simulink model "quhua"  (Simulink 6.3)
settings: Solver=ode45  StartTime=0.0  StopTime=0.08  RelTol=1e-3
settings Model: LastModifiedBy=Administrator

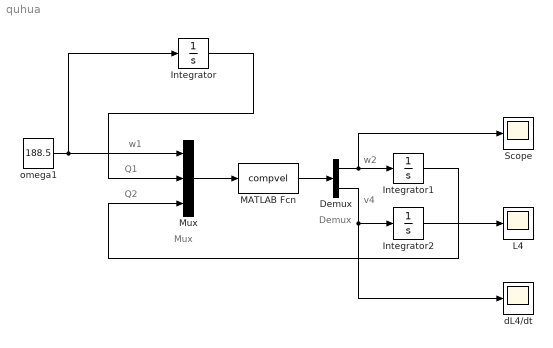
== system quhua ==
  note: Mux
  note: Demux
  note: w1
  note: Q1
  note: Q2
  note: w2
  note: v4
  Demux : Demux  Outputs=2
  Integrator : Integrator
  Integrator1 : Integrator
  Integrator2 : Integrator
  L4 : Scope
      settings: TimeRange=0.08  YMin=-60  YMax=0
  MATLAB Fcn : MATLABFcn  MATLABFcn=compvel
  Mux : Mux  Inputs=3
  Scope : Scope
  dL4/dt : Scope
      settings: SaveName=ScopeData2
  omega1 : Constant  Value=188.5
  wires:
  omega1/1 -> Mux/1, Integrator/1
  Integrator/1 -> Mux/2
  Mux/1 -> MATLAB Fcn/1
  MATLAB Fcn/1 -> Demux/1
  Demux/1 -> Scope/1, Integrator1/1
  Demux/2 -> Integrator2/1, dL4/dt/1
  Integrator1/1 -> Mux/3
  Integrator2/1 -> L4/1
